simulink model "pid_thuchanh"  (R2023b)
settings: Solver=VariableStepAuto  StartTime=0.0  StopTime=100  FixedStep=0.01  RelTol=1e-3
InitFcn:
  | para
values from neighbouring files (symbols this model uses):
  a = 1    [para.m]
  b = -1    [para.m]
  c = 0.5    [para.m]
  d_threshold = 0.2    [para.m]
  J = 0.0025    [para.m]
  Ke = 0.05    [para.m]
  Kt = 0.05    [para.m]
  L = 0.005    [para.m]
  R = 2    [para.m]
libraries: slpidlib x2
settings Model: Creator=Administrator  LastModifiedBy=hongquan

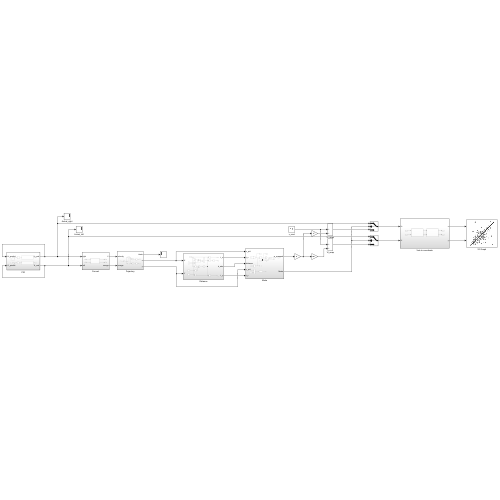
[thumbnail: Simulink's stored preview of the top-level diagram]
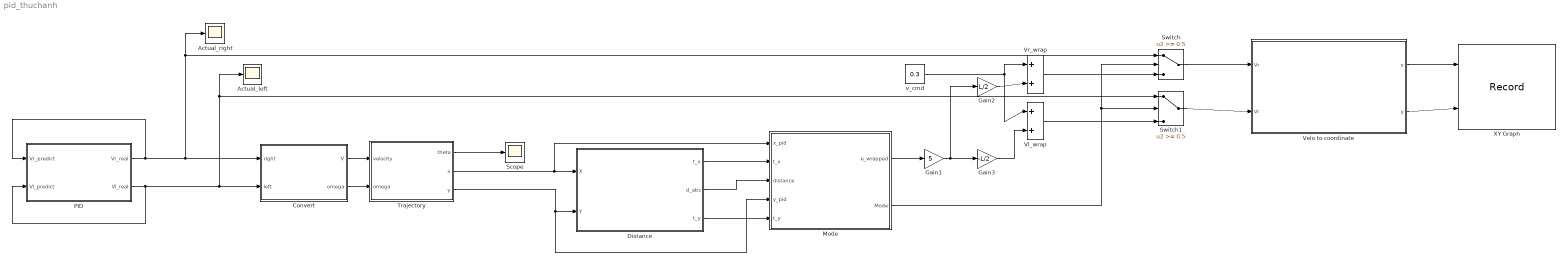
== system pid_thuchanh ==
  Actual_left : Scope
  Actual_right : Scope
  Convert : Subsystem
  Distance : Subsystem
  Gain1 : Gain  Gain=5
  Gain2 : Gain  Gain=L/2
  Gain3 : Gain  Gain=-L/2
  Mode : Subsystem
  PID : Subsystem
  Scope : Scope
  Switch : Switch  Threshold=0.5  SaturateOnIntegerOverflow=off  InputSameDT=off
  Switch1 : Switch  Threshold=0.5  SaturateOnIntegerOverflow=off  InputSameDT=off
  Trajectory : Subsystem
  Velo to coordinate : Subsystem
  Vl_wrap : Sum  Inputs=|++
  Vr_wrap : Sum  Inputs=|++
  XY Graph : Record  FileSettingsInternal="{\"entries\":[{\"content\":{\"excelSettings\":{\"content\":{},\"type\":\"Streamout.ExcelSettings\"}},\"type\":\"Streamout.FileSettingStorage\",\"uuid\":\"\"}],\"packageUris\":[\"http:\\/\\/schema.mathworks.com\\/mf0\\/streamout_blocks\\/R2020a\"],\"version\":\"1.0\"}"  Layout=[1 1]  SignalsInternal="{\"entries\":[{\"content\":{\"signals\":[{\"content\":{\"blockPath\":[],\"dimensions\":[1],\"domain\":\"\",\"lineColor\":\"#a2142f\",\"plots\":[1],\"port\":1,\"signalID\":8,\"signalName\":\"Velo to coordinate:1\"},\"type\":\"RecordBlkView.Signal\",\"uuid\":\"\"},{\"content\":{\"blockPath\":[],\"dimensions\":[1],\"domain\":\"\",\"lineColor\":\"#139fff\",\"plots\":[1],\"port\":2,\"signalID\":11,\"signalName\":\"Velo to coordinate:2\"},\"type\":\"RecordBlkView.Signal\",\"uuid\":\"\"}]},\"type\":\"RecordBlkView.InputSignals\",\"uuid\":\"\"}],\"packageUris\":[\"http:\\/\\/schema.mathworks.com\\/mf0\\/streamout_blocks\\/R2020a\"],\"version\":\"1.0\"}"  VisualizationBindings="{\"xyplotplugin\":{\"info\":[{\"series\":[{\"bindingParametersList\":[{\"parameter\":\"X-Axis\",\"signalID\":8,\"signalName\":\"Velo to coordinate:1\"},{\"parameter\":\"Y-Axis\",\"signalID\":11,\"signalName\":\"Velo to coordinate:2\"}],\"seriesID\":11598}],\"subplotID\":1}]}}"  CompatibilityTag=XY
  v_cmd : Constant  Value=0.3
  wires:
  PID/1(Vr_real) -> Switch/1, Actual_right/1, Convert/1(right), PID/1(Vr_predict)
  PID/2(Vl_real) -> PID/2(Vl_predict), Convert/2(left), Switch1/1, Actual_left/1
  Trajectory/3(y) -> Mode/4(y_pid), Distance/2(Y)
  Trajectory/2(x) -> Distance/1(X), Mode/1(x_pid)
  Convert/1(V) -> Trajectory/1(velocity)
  Convert/2(omega) -> Trajectory/2(omega)
  Distance/1(t_x) -> Mode/2(t_x)
  Distance/3(t_y) -> Mode/5(t_y)
  Mode/1(e_wrapped) -> Gain1/1
  Gain1/1 -> Gain2/1, Gain3/1
  Velo to coordinate/1(x) -> XY Graph/1
  Gain2/1 -> Vr_wrap/2
  v_cmd/1 -> Vl_wrap/1, Vr_wrap/1
  Gain3/1 -> Vl_wrap/2
  Vr_wrap/1 -> Switch/3
  Vl_wrap/1 -> Switch1/3
  Switch/1 -> Velo to coordinate/1(Vr)
  Switch1/1 -> Velo to coordinate/2(Vl)
  Velo to coordinate/2(y) -> XY Graph/2
  Mode/2(Mode) -> Switch/2, Switch1/2
  Distance/2(d_abs) -> Mode/3(distance)
  Trajectory/1(theta) -> Scope/1

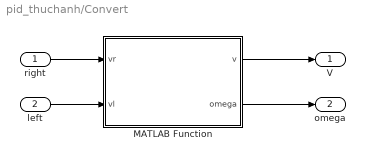
== system pid_thuchanh/Convert ==
  right : Inport
  left : Inport  Port=2
  MATLAB Function : MATLAB Function  TreatAsAtomicUnit=on
  V : Outport
  omega : Outport  Port=2
  wires:
  left/1 -> MATLAB Function/2(vl)
  right/1 -> MATLAB Function/1(vr)
  MATLAB Function/1(v) -> V/1
  MATLAB Function/2(omega) -> omega/1

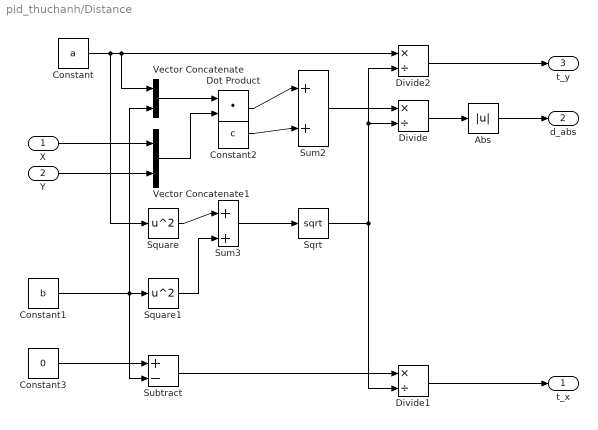
== system pid_thuchanh/Distance ==
  X : Inport
  Y : Inport  Port=2
  Abs : Abs  SaturateOnIntegerOverflow=off
  Constant : Constant  Value=a
  Constant1 : Constant  Value=b
  Constant2 : Constant  Value=c
  Constant3 : Constant  Value=0
  Divide : Product  Inputs=*/
  Divide1 : Product  Inputs=*/
  Divide2 : Product  Inputs=*/
  Dot Product : DotProduct  OutDataTypeStr=Inherit: Inherit via internal rule
  Sqrt : Sqrt
  Square : Math  Operator=square
  Square1 : Math  Operator=square
  Subtract : Sum  Inputs=+-
  Sum2 : Sum  Inputs=|++
  Sum3 : Sum  Inputs=|++
  Vector Concatenate : Concatenate
  Vector Concatenate1 : Concatenate
  t_x : Outport
  d_abs : Outport  Port=2
  t_y : Outport  Port=3
  wires:
  Divide/1 -> Abs/1
  Constant/1 -> Square/1, Vector Concatenate/1, Divide2/1
  Constant1/1 -> Vector Concatenate/2, Subtract/2, Square1/1
  Y/1 -> Vector Concatenate1/2
  X/1 -> Vector Concatenate1/1
  Subtract/1 -> Divide1/1
  Vector Concatenate/1 -> Dot Product/1
  Constant3/1 -> Subtract/1
  Vector Concatenate1/1 -> Dot Product/2
  Square/1 -> Sum3/1
  Abs/1 -> d_abs/1
  Square1/1 -> Sum3/2
  Dot Product/1 -> Sum2/1
  Constant2/1 -> Sum2/2
  Sum3/1 -> Sqrt/1
  Sum2/1 -> Divide/1
  Sqrt/1 -> Divide2/2, Divide/2, Divide1/2
  Divide2/1 -> t_y/1
  Divide1/1 -> t_x/1

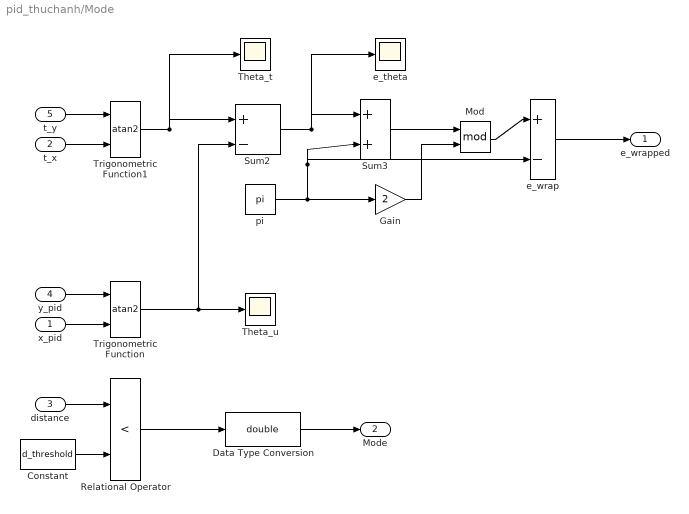
== system pid_thuchanh/Mode ==
  x_pid : Inport
  t_x : Inport  Port=2
  distance : Inport  Port=3
  y_pid : Inport  Port=4
  t_y : Inport  Port=5
  Constant : Constant  Value=d_threshold
  Data Type Conversion : DataTypeConversion  OutDataTypeStr=double  SaturateOnIntegerOverflow=off  RndMeth=Floor
  Gain : Gain  Gain=2
  Mod : Math  Operator=mod
  Relational Operator : RelationalOperator  Operator=<  OutDataTypeStr=boolean  RndMeth=Simplest  InputSameDT=off
  Sum2 : Sum  Inputs=|+-
  Sum3 : Sum  Inputs=|++
  Theta_t : Scope
  Theta_u : Scope
  Trigonometric Function : Trigonometry  Operator=atan2
  Trigonometric Function1 : Trigonometry  Operator=atan2
  e_theta : Scope
  e_wrap : Sum  Inputs=|+-
  pi : Constant  Value=pi
  e_wrapped : Outport
  Mode : Outport  Port=2
  wires:
  t_y/1 -> Trigonometric Function1/1
  Trigonometric Function/1 -> Theta_u/1, Sum2/2
  Trigonometric Function1/1 -> Theta_t/1, Sum2/1
  Constant/1 -> Relational Operator/2
  t_x/1 -> Trigonometric Function1/2
  distance/1 -> Relational Operator/1
  y_pid/1 -> Trigonometric Function/1
  x_pid/1 -> Trigonometric Function/2
  Relational Operator/1 -> Data Type Conversion/1
  Sum2/1 -> e_theta/1, Sum3/1
  pi/1 -> Sum3/2, e_wrap/2, Gain/1
  Data Type Conversion/1 -> Mode/1
  Sum3/1 -> Mod/1
  Gain/1 -> Mod/2
  Mod/1 -> e_wrap/1
  e_wrap/1 -> e_wrapped/1

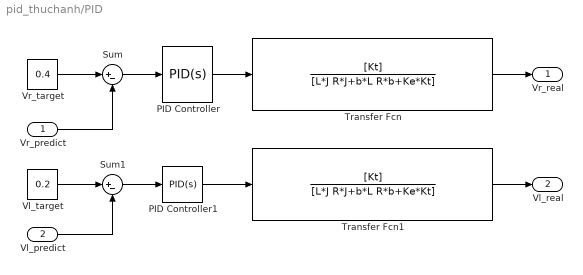
== system pid_thuchanh/PID ==
  Vr_predict : Inport
  Vl_predict : Inport  Port=2
  PID Controller : slpidlib/PID Controller  Controller=PID  Form=Parallel  TimeDomain=Continuous-time  UseExternalTs=off  SampleTime=-1  IntegratorMethod=Forward Euler  FilterMethod=Forward Euler  ControllerParametersSource=internal  P=1  I=1  UseKiTs=off  D=0  N=100  UseFilter=on  TunerSelectOption=Transfer Function Based (PID Tuner App)  InitialConditionSource=internal  InitialConditionForIntegrator=0  InitialConditionForFilter=0  DifferentiatorICPrevScaledInput=0  ExternalReset=none  TrackingMode=off  Kt=1  LimitOutput=off  SatLimitsSource=internal  UpperSaturationLimit=inf  LowerSaturationLimit=-inf  LinearizeAsGain=on  AntiWindupMode=none  Kb=1  LimitIntegrator=off  UpperIntegratorSaturationLimit=inf  LowerIntegratorSaturationLimit=-inf  POutMin=[]  POutMax=[]  IOutMin=[]  IOutMax=[]  DOutMin=[]  DOutMax=[]  NOutMin=[]  NOutMax=[]  SumOutMin=[]  SumOutMax=[]  SaturationOutMin=[]  SaturationOutMax=[]  PParamMin=[]  PParamMax=[]  IParamMin=[]  IParamMax=[]  DParamMin=[]  DParamMax=[]  NParamMin=[]  NParamMax=[]  KbParamMin=[]  KbParamMax=[]  KtParamMin=[]  KtParamMax=[]  KbOutMin=[]  KbOutMax=[]  KtOutMin=[]  KtOutMax=[]  IntegratorOutMin=[]  IntegratorOutMax=[]  FilterOutMin=[]  FilterOutMax=[]  SumI1OutMin=[]  SumI1OutMax=[]  SumI2OutMin=[]  SumI2OutMax=[]  SumI3OutMin=[]  SumI3OutMax=[]  SumI4OutMin=[]  SumI4OutMax=[]  SumDOutMin=[]  SumDOutMax=[]  DifferentiatorOutMin=[]  DifferentiatorOutMax=[]  FilterDiffOutCoefMin=[]  FilterDiffOutCoefMax=[]  ReciprocalOutMin=[]  ReciprocalOutMax=[]  SumDenOutMin=[]  SumDenOutMax=[]  SumNumOutMin=[]  SumNumOutMax=[]  DivideOutMin=[]  DivideOutMax=[]  UdiffTsProdOutMin=[]  UdiffTsProdOutMax=[]  NTsProdOutMin=[]  NTsProdOutMax=[]  UintegralTsProdOutMin=[]  UintegralTsProdOutMax=[]  UngainTsProdOutMin=[]  UngainTsProdOutMax=[]  ClampingZeroOutDataTypeStr=Inherit: Inherit via back propagation  ClampingZeroOutMin=[]  ClampingZeroOutMax=[]  FilterDenConstantOutDataTypeStr=Inherit: Inherit via back propagation  FilterDenConstantOutMin=[]  FilterDenConstantOutMax=[]  PCopyOutDataTypeStr=Inherit: Inherit via back propagation  PCopyOutMin=[]  PCopyOutMax=[]  NCopyOutDataTypeStr=Inherit: Inherit via back propagation  NCopyOutMin=[]  NCopyOutMax=[]  IntegratorContinuousStateAttributes=''  IntegratorStateMustResolveToSignalObject=off  IntegratorRTWStateStorageClass=Auto  FilterContinuousStateAttributes=''  FilterStateMustResolveToSignalObject=off  FilterRTWStateStorageClass=Auto  ParallelPVariant=InternalParameters  IdealPVariant=Disabled  IVariant=InternalParameters  DVariant=InternalParameters  IntegratorVariant=Continuous  SatVariant=Disabled  AWVariant=Passthrough  PCopyVariant=Disabled  TRVariant=Disabled  FdbkBlocksVariant=Forward  IdealPFdbkVariant=Disabled  SatFdbkVariant=Disabled  DerivativeFilterVariant=ContFilter  NVariant=InternalParameters  NCopyVariant=Disabled  FilterICVariant=InternalICsFilter  IntegratorICVariant=InternalICs  ExternalResetVariant=Disabled  TRSumVariant=Passthrough  SumFdbkVariant=Disabled  SumVariant=Sum_PID  TsampFilterVariant=InternalTs  TsampNgainVariant=Passthrough  TsampIntegralVariant=Disabled_SignalSpec  ExternalSaturationOutDataTypeStr=Inherit: Same as second input
  PID Controller1 : slpidlib/PID Controller  Controller=PID  Form=Parallel  TimeDomain=Continuous-time  UseExternalTs=off  SampleTime=-1  IntegratorMethod=Forward Euler  FilterMethod=Forward Euler  ControllerParametersSource=internal  P=1  I=1  UseKiTs=off  D=0  N=100  UseFilter=on  TunerSelectOption=Transfer Function Based (PID Tuner App)  InitialConditionSource=internal  InitialConditionForIntegrator=0  InitialConditionForFilter=0  DifferentiatorICPrevScaledInput=0  ExternalReset=none  TrackingMode=off  Kt=1  LimitOutput=off  SatLimitsSource=internal  UpperSaturationLimit=inf  LowerSaturationLimit=-inf  LinearizeAsGain=on  AntiWindupMode=none  Kb=1  LimitIntegrator=off  UpperIntegratorSaturationLimit=inf  LowerIntegratorSaturationLimit=-inf  POutMin=[]  POutMax=[]  IOutMin=[]  IOutMax=[]  DOutMin=[]  DOutMax=[]  NOutMin=[]  NOutMax=[]  SumOutMin=[]  SumOutMax=[]  SaturationOutMin=[]  SaturationOutMax=[]  PParamMin=[]  PParamMax=[]  IParamMin=[]  IParamMax=[]  DParamMin=[]  DParamMax=[]  NParamMin=[]  NParamMax=[]  KbParamMin=[]  KbParamMax=[]  KtParamMin=[]  KtParamMax=[]  KbOutMin=[]  KbOutMax=[]  KtOutMin=[]  KtOutMax=[]  IntegratorOutMin=[]  IntegratorOutMax=[]  FilterOutMin=[]  FilterOutMax=[]  SumI1OutMin=[]  SumI1OutMax=[]  SumI2OutMin=[]  SumI2OutMax=[]  SumI3OutMin=[]  SumI3OutMax=[]  SumI4OutMin=[]  SumI4OutMax=[]  SumDOutMin=[]  SumDOutMax=[]  DifferentiatorOutMin=[]  DifferentiatorOutMax=[]  FilterDiffOutCoefMin=[]  FilterDiffOutCoefMax=[]  ReciprocalOutMin=[]  ReciprocalOutMax=[]  SumDenOutMin=[]  SumDenOutMax=[]  SumNumOutMin=[]  SumNumOutMax=[]  DivideOutMin=[]  DivideOutMax=[]  UdiffTsProdOutMin=[]  UdiffTsProdOutMax=[]  NTsProdOutMin=[]  NTsProdOutMax=[]  UintegralTsProdOutMin=[]  UintegralTsProdOutMax=[]  UngainTsProdOutMin=[]  UngainTsProdOutMax=[]  ClampingZeroOutDataTypeStr=Inherit: Inherit via back propagation  ClampingZeroOutMin=[]  ClampingZeroOutMax=[]  FilterDenConstantOutDataTypeStr=Inherit: Inherit via back propagation  FilterDenConstantOutMin=[]  FilterDenConstantOutMax=[]  PCopyOutDataTypeStr=Inherit: Inherit via back propagation  PCopyOutMin=[]  PCopyOutMax=[]  NCopyOutDataTypeStr=Inherit: Inherit via back propagation  NCopyOutMin=[]  NCopyOutMax=[]  IntegratorContinuousStateAttributes=''  IntegratorStateMustResolveToSignalObject=off  IntegratorRTWStateStorageClass=Auto  FilterContinuousStateAttributes=''  FilterStateMustResolveToSignalObject=off  FilterRTWStateStorageClass=Auto  ParallelPVariant=InternalParameters  IdealPVariant=Disabled  IVariant=InternalParameters  DVariant=InternalParameters  IntegratorVariant=Continuous  SatVariant=Disabled  AWVariant=Passthrough  PCopyVariant=Disabled  TRVariant=Disabled  FdbkBlocksVariant=Forward  IdealPFdbkVariant=Disabled  SatFdbkVariant=Disabled  DerivativeFilterVariant=ContFilter  NVariant=InternalParameters  NCopyVariant=Disabled  FilterICVariant=InternalICsFilter  IntegratorICVariant=InternalICs  ExternalResetVariant=Disabled  TRSumVariant=Passthrough  SumFdbkVariant=Disabled  SumVariant=Sum_PID  TsampFilterVariant=InternalTs  TsampNgainVariant=Passthrough  TsampIntegralVariant=Disabled_SignalSpec  ExternalSaturationOutDataTypeStr=Inherit: Same as second input
  Sum : Sum  Inputs=|+-
  Sum1 : Sum  Inputs=|+-
  Transfer Fcn : TransferFcn  Numerator=[Kt]  Denominator=[L*J R*J+b*L R*b+Ke*Kt]
  Transfer Fcn1 : TransferFcn  Numerator=[Kt]  Denominator=[L*J R*J+b*L R*b+Ke*Kt]
  Vl_target : Constant  Value=0.2
  Vr_target : Constant  Value=0.4
  Vr_real : Outport
  Vl_real : Outport  Port=2
  wires:
  Vl_predict/1 -> Sum1/2
  Vl_target/1 -> Sum1/1
  Vr_target/1 -> Sum/1
  Vr_predict/1 -> Sum/2
  Sum/1 -> PID Controller/1
  Sum1/1 -> PID Controller1/1
  PID Controller1/1 -> Transfer Fcn1/1
  PID Controller/1 -> Transfer Fcn/1
  Transfer Fcn/1 -> Vr_real/1
  Transfer Fcn1/1 -> Vl_real/1

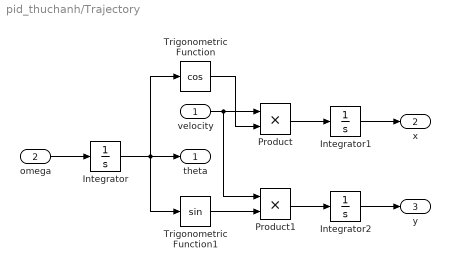
== system pid_thuchanh/Trajectory ==
  velocity : Inport
  omega : Inport  Port=2
  Integrator : Integrator
  Integrator1 : Integrator
  Integrator2 : Integrator
  Product : Product
  Product1 : Product
  Trigonometric Function : Trigonometry  Operator=cos
  Trigonometric Function1 : Trigonometry
  theta : Outport
  x : Outport  Port=2
  y : Outport  Port=3
  wires:
  Product1/1 -> Integrator2/1
  omega/1 -> Integrator/1
  velocity/1 -> Product/1, Product1/1
  Integrator/1 -> Trigonometric Function/1, theta/1, Trigonometric Function1/1
  Trigonometric Function1/1 -> Product1/2
  Trigonometric Function/1 -> Product/2
  Product/1 -> Integrator1/1
  Integrator1/1 -> x/1
  Integrator2/1 -> y/1

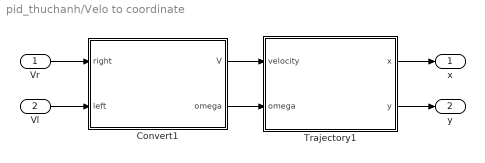
== system pid_thuchanh/Velo to coordinate ==
  Vr : Inport
  Vl : Inport  Port=2
  Convert1 : Subsystem
  Trajectory1 : Subsystem
  x : Outport
  y : Outport  Port=2
  wires:
  Convert1/2(omega) -> Trajectory1/2(omega)
  Vr/1 -> Convert1/1(right)
  Convert1/1(V) -> Trajectory1/1(velocity)
  Vl/1 -> Convert1/2(left)
  Trajectory1/2(y) -> y/1
  Trajectory1/1(x) -> x/1

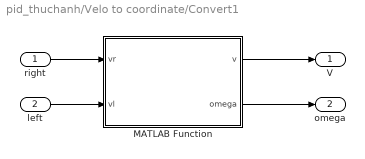
== system pid_thuchanh/Velo to coordinate/Convert1 ==
  right : Inport
  left : Inport  Port=2
  MATLAB Function : MATLAB Function  TreatAsAtomicUnit=on
  V : Outport
  omega : Outport  Port=2
  wires:
  left/1 -> MATLAB Function/2(vl)
  right/1 -> MATLAB Function/1(vr)
  MATLAB Function/1(v) -> V/1
  MATLAB Function/2(omega) -> omega/1

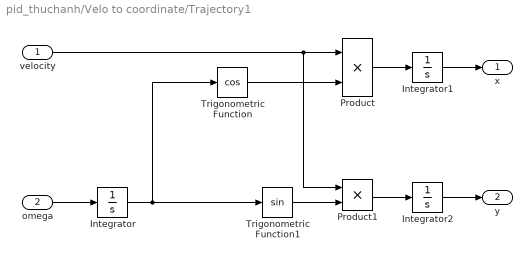
== system pid_thuchanh/Velo to coordinate/Trajectory1 ==
  velocity : Inport
  omega : Inport  Port=2
  Integrator : Integrator
  Integrator1 : Integrator
  Integrator2 : Integrator
  Product : Product
  Product1 : Product
  Trigonometric Function : Trigonometry  Operator=cos
  Trigonometric Function1 : Trigonometry
  x : Outport
  y : Outport  Port=2
  wires:
  Product1/1 -> Integrator2/1
  omega/1 -> Integrator/1
  velocity/1 -> Product1/1, Product/1
  Integrator/1 -> Trigonometric Function1/1, Trigonometric Function/1
  Trigonometric Function1/1 -> Product1/2
  Trigonometric Function/1 -> Product/2
  Product/1 -> Integrator1/1
  Integrator1/1 -> x/1
  Integrator2/1 -> y/1

== matlab function pid_thuchanh/Convert/MATLAB Function ==
  data: vr input; v output; vl input; omega output
function [v, omega] = computeVels(vr, vl)
    L = 0.2; % khoảng cách giữa hai bánh (m)
    v = (vr + vl)/2;
    omega = (vr - vl)/L;
end

== matlab function pid_thuchanh/Velo to coordinate/Convert1/MATLAB Function ==
  data: vr input; v output; vl input; omega output
function [v, omega] = computeVels(vr, vl)
    L = 0.2; % khoảng cách giữa hai bánh (m)
    v = (vr + vl)/2;
    omega = (vr - vl)/L;
end
